simulink model "P4_SLX"  (R2024a)
settings: Solver=ode3  StartTime=0.0  StopTime=inf  FixedStep=Ts  RelTol=1e-3
PostLoadFcn:
  | try
  | if isempty(which('ZHAWcbfcn'));
  | callback_fid07124=fopen('ZHAWcbfcn.m','w');
  | [~]=fprintf(callback_fid07124,'%s',get_param([bdroot,'/ Setup SLDRT'],'ClipboardFcn'));
  | [~]=fclose(callback_fid07124);
  | setpref('ZHAW_SLDRT_lib','cb_fcn',which('ZHAWcbfcn'))
  | clear callback_fid07124
  | end
  | catch
  | clear callback_fid07124
  | end
  | Ts=eval(get_param([bdroot,'/ Setup SLDRT'],'Ts'));
InitFcn:
  | Ts=eval(get_param([bdroot,'/ Setup SLDRT'],'Ts'));
undefined symbols (not defined in the file or in its folder): National_Instruments, PCIe
libraries: sldrtlib x3, cstblocks x2
(part 2 of 2)

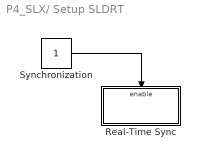
== system P4_SLX/ Setup SLDRT ==
  Real-Time Sync : Subsystem
  Synchronization : Constant
  wires:
  Synchronization/1 -> Real-Time Sync/Enable

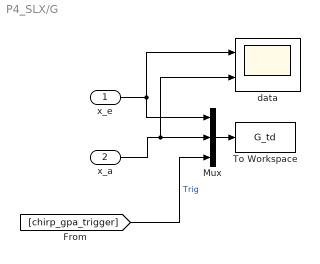
== system P4_SLX/G ==
  x_e : Inport
  x_a : Inport  Port=2
  Mux : Mux  Inputs=3
  To Workspace : ToWorkspace  VariableName=G_td  SaveFormat=Structure With Time  SampleTime=Ts
  data : Scope  NumInputPorts=2
      settings: CopyFcn=try ZHAWcbfcn('copyScope'); end  NameChangeFcn=try ZHAWcbfcn('namechangeScope'); end
  wires:
  x_e/1 -> data/1, Mux/1
  x_a/1 -> data/2, Mux/2
  Mux/1 -> To Workspace/1
  [chirp_gpa_trigger] -> Mux/3  "Trig"

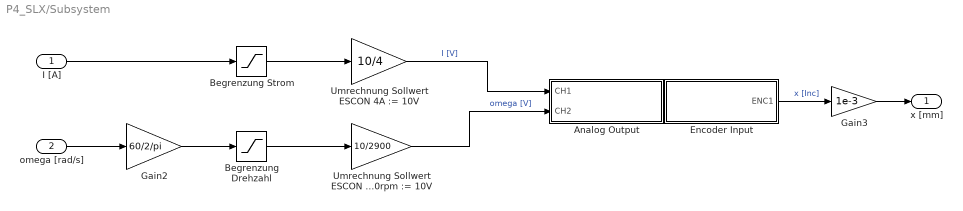
== system P4_SLX/Subsystem ==
  I [A] : Inport
  omega [rad/s] : Inport  Port=2
  Analog Output : Subsystem  mask(NI Analog Output){device=PCIe-6321, connect=Banana Terminal, ch1=on, ch2=on, ch3=off, ch4=off, Ts=Ts}
      mask prompts: device "NI Device Type:"; connect "Connector Box :"; Ts "Sample Time:"
      mask help:
      | DA Converter
      | +/- 10V
      mask init:
      | try ch_list = ZHAWcbfcn('get_ch_list'); end
      | try ZHAWcbfcn('BlockUpdate'); end
      settings: OpenFcn=try ZHAWcbfcn('openMask'); end
      settings: CopyFcn=|
      | try
      | ZHAWcbfcn('CopyIOblock')
      | end
      | set_param(gcb,'OpenFcn','try ZHAWcbfcn(''openMask''); end')
      mask TypeOptions device: PCI-6221 | PCI-6259 | PCIe-6259 | PCIe-6321 | PCIe-6363
      mask Callback device:
      | try ZHAWcbfcn('SetChannelNumber'); end
      | try ZHAWcbfcn('SetConnectorBox'); end
      mask TypeOptions connect: BNC Terminal | Banana Terminal | Screw Terminal
      mask Callback connect: try ZHAWcbfcn('SetConnectorBox'); end
      mask DialogControl DescGroupVar Prompt: NI Analog Output (R2024a)
      mask Display: disp('NI\nPCIe-6321')
  Begrenzung Drehzahl : Saturate  UpperLimit=2900  LowerLimit=-2900
  Begrenzung Strom : Saturate
  Encoder Input : Subsystem  mask(NI Encoder Input){device=PCIe-6321, connect=Banana Terminal, reset=off, ch1=on, ch2=off, ch3=off, ch4=off, Ts=Ts}
      mask prompts: device "NI Device Type:"; connect "Connector Box:"; reset "Reset at Index:"; ch1 "ENC1"; ch2 "ENC2"; ch3 "ENC3"; ch4 "ENC4"; Ts "Sample Time:"
      mask help:
      | Quadratur Encoder.
      | X4 Decoding.
      | Output is increments.
      mask init:
      | try ch_list = ZHAWcbfcn('get_ch_list'); end
      | try ZHAWcbfcn('BlockUpdate'); end
      settings: AttributesFormatString=Index Reset: %<reset>  OpenFcn=try ZHAWcbfcn('openMask'); end
      settings: CopyFcn=|
      | try
      | ZHAWcbfcn('CopyIOblock')
      | end
      | set_param(gcb,'OpenFcn','try ZHAWcbfcn(''openMask''); end')
      mask TypeOptions device: PCI-6221 | PCI-6259 | PCIe-6259 | PCIe-6321 | PCIe-6363
      mask Callback device: try ZHAWcbfcn('SetChannelNumber'); end
      mask TypeOptions connect: BNC Terminal | Banana Terminal | Screw Terminal
      mask Callback connect: try ZHAWcbfcn('SetConnectorBox'); end
      mask TypeOptions reset: on | off
      mask Callback reset: try ZHAWcbfcn('SetEncoderReset'); end
      mask DialogControl DescGroupVar Prompt: NI Encoder Input (R2024a)
      mask Display: disp('NI\nPCIe-6321')
  Gain2 : Gain  Gain=60/2/pi
  Gain3 : Gain  Gain=1e-3
  Umrechnung Sollwert ESCON 2900rpm := 10V : Gain  Gain=10/2900
  Umrechnung Sollwert ESCON 4A := 10V : Gain  Gain=10/4
  x [mm] : Outport
  wires:
  Gain3/1 -> x [mm]/1
  I [A]/1 -> Begrenzung Strom/1
  Begrenzung Strom/1 -> Umrechnung Sollwert ESCON 4A := 10V/1
  Umrechnung Sollwert ESCON 4A := 10V/1 -> Analog Output/1(CH1)  "I [V]"
  omega [rad/s]/1 -> Gain2/1
  Gain2/1 -> Begrenzung Drehzahl/1
  Begrenzung Drehzahl/1 -> Umrechnung Sollwert ESCON 2900rpm := 10V/1
  Umrechnung Sollwert ESCON 2900rpm := 10V/1 -> Analog Output/2(CH2)  "omega [V]"
  Encoder Input/1(ENC1) -> Gain3/1  "x [Inc]"

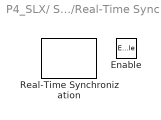
== system P4_SLX/ Setup SLDRT/Real-Time Sync ==
  Enable : EnablePort
  Real-Time Synchronization : sldrtlib/Real-Time Synchronization  SampleTime=Ts  MaxMissedTicks=inf  ShowMissedTicks=off  YieldWhenWaiting=off

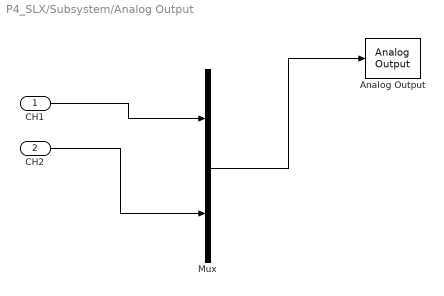
== system P4_SLX/Subsystem/Analog Output ==
  CH1 : Inport
  CH2 : Inport  Port=2
  Analog Output : sldrtlib/Analog Output  SampleTime=Ts  MaxMissedTicks=10  ShowMissedTicks=off  YieldWhenWaiting=off  DrvName=National_Instruments/PCIe-6321  DrvAddress=4294967295  DrvOptions="[1  0  0  2  2  2  2]"  Channels=ch_list  RangeMode=1  VoltRange=1  InitialValue=0  FinalValue=0
      settings: AttributesFormatString=National Instruments\nPCIe-6321 [auto]
  Mux : Mux  Inputs=2
  wires:
  Mux/1 -> Analog Output/1
  CH1/1 -> Mux/1
  CH2/1 -> Mux/2

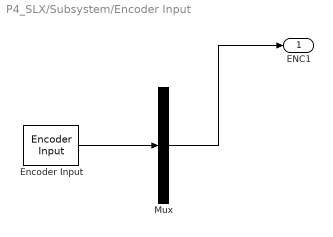
== system P4_SLX/Subsystem/Encoder Input ==
  Encoder Input : sldrtlib/Encoder Input  SampleTime=Ts  MaxMissedTicks=10  ShowMissedTicks=off  YieldWhenWaiting=off  DrvName=National_Instruments/PCIe-6321  DrvAddress=4294967295  DrvOptions="[1  0  0  2  2  2  2]"  Channels=ch_list  QuadMode=3  IndexPulse=1  InputFilter=Inf  DataType=1
      settings: AttributesFormatString=National Instruments\nPCIe-6321 [auto]
  Mux : Demux  Outputs=1
  ENC1 : Outport  VectorParamsAs1DForOutWhenUnconnected=off
  wires:
  Encoder Input/1 -> Mux/1
  Mux/1 -> ENC1/1
